simulink model "piController"  (R2024a)
settings: Solver=VariableStepAuto  StartTime=0.0  StopTime=20  RelTol=1e-3
values from neighbouring files (symbols this model uses):
  rotationSpeedControl = 300    [plotPiController.m]
undefined symbols (not defined in the file or in its folder): TN
settings Model: Creator=janho  LastModifiedBy=janho

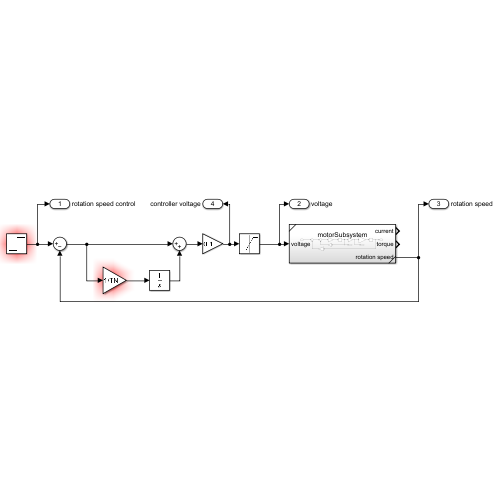
[thumbnail: Simulink's stored preview of the top-level diagram]
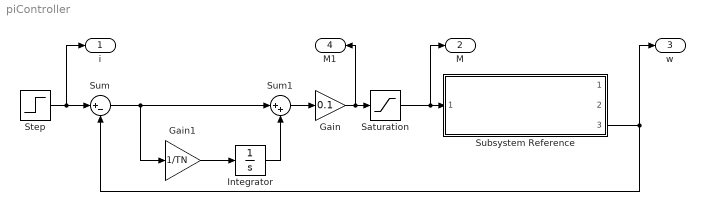
== system piController ==
  Gain : Gain  Gain=0.1
  Gain1 : Gain  Gain=1/TN
  Integrator : Integrator
  Saturation : Saturate  UpperLimit=10  LowerLimit=-10
  Step : Step  Time=0  After=rotationSpeedControl  SampleTime=0
  Subsystem Reference : Subsystem  ReferencedSubsystem=motorSubsystem
  Sum : Sum  Inputs=|+-
  Sum1 : Sum  Inputs=|++
  i : Outport  SignalName=rotation speed control
  M : Outport  Port=2  SignalName=voltage
  w : Outport  Port=3  SignalName=rotation speed
  M1 : Outport  Port=4  SignalName=controller voltage
  wires:
  Sum/1 -> Sum1/1, Gain1/1
  Step/1 -> i/1, Sum/1
  Saturation/1 -> M/1, Subsystem Reference/1
  Subsystem Reference/3 -> w/1, Sum/2
  Integrator/1 -> Sum1/2
  Gain1/1 -> Integrator/1
  Sum1/1 -> Gain/1
  Gain/1 -> M1/1, Saturation/1
